simulink model "Virtual_Exhaust_Aftertreatment_Controller"  (R2016b)
settings: Solver=FixedStepDiscrete  StartTime=0.0  StopTime=inf  FixedStep=VirtExhATCtrlr.tiSimnTiStep_C  RelTol=1e-3  EnableMultiTasking=on
settings Model: Creator=m01wolf  LastModifiedBy=bunver
settings DataIOCC: SaveFormat=StructureWithTime  SaveOutput=off  DSMLogging=off  VisualizeSimOutput=off  SaveTime=off  SignalLoggingName=Results
settings OptimizationCC: BlockReduction=off  ConditionallyExecuteInputs=off  LifeSpan=inf
settings DebuggingCC: AllowSymbolicDim=off  SFUnexpectedBacktrackingDiag=warning  SFNoUnconditionalDefaultTransitionDiag=warning  SFExecutionAtInitializationDiag=none
settings ModelReferenceCC: ModelReferenceNumInstancesAllowed=Single  PropagateSignalLabelsOutOfModel=off
settings GRTTargetCC: TargetLangStandard=C89/C90 (ANSI)
settings ConfigComp: CovMetricSettings=dw  CovHtmlReporting=on  CovSaveCumulativeToWorkspaceVar=on  CovSaveSingleToWorkspaceVar=on  CovExternalEMLEnable=off

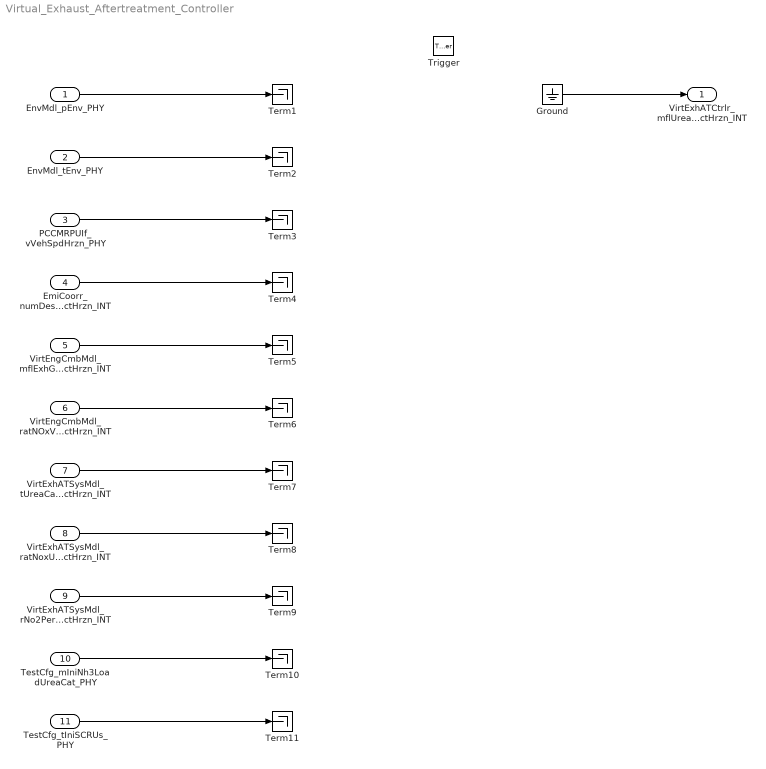
== system Virtual_Exhaust_Aftertreatment_Controller ==
  EnvMdl_pEnv_PHY : Inport
  EnvMdl_tEnv_PHY : Inport  Port=2
  PCCMRPUIf_vVehSpdHrzn_PHY : Inport  Port=3  PortDimensions=VirtExhATCtrlr_numHrznSize_CA
  EmiCoorr_numDesEngOperModVectHrzn_INT : Inport  Port=4  PortDimensions=VirtExhATCtrlr_numHrznSize_CA
  VirtEngCmbMdl_mflExhGasVectHrzn_INT : Inport  Port=5  PortDimensions=VirtExhATCtrlr_numHrznSize_CA
  VirtEngCmbMdl_ratNOxVectHrzn_INT : Inport  Port=6  PortDimensions=VirtExhATCtrlr_numHrznSize_CA
  VirtExhATSysMdl_tUreaCatUsVectHrzn_INT : Inport  Port=7  PortDimensions=VirtExhATCtrlr_numHrznSize_CA
  VirtExhATSysMdl_ratNoxUreaCatDsVectHrzn_INT : Inport  Port=8  PortDimensions=VirtExhATCtrlr_numHrznSize_CA
  VirtExhATSysMdl_rNo2PerNoxUreaCatUsVectHrzn_INT : Inport  Port=9  PortDimensions=VirtExhATCtrlr_numHrznSize_CA
  TestCfg_mIniNh3LoadUreaCat_PHY : Inport  Port=10
  TestCfg_tIniSCRUs_PHY : Inport  Port=11
  Trigger : TriggerPort  TriggerType=function-call  VariantControl=Variant  PortDimensions=1
  Ground : Ground
  Term{1..11} (11 alike) : Terminator
  VirtExhATCtrlr_mflUreaDesVectHrzn_INT : Outport  PortDimensions=VirtExhATCtrlr_numHrznSize_CA
  wires:
  Ground/1 -> VirtExhATCtrlr_mflUreaDesVectHrzn_INT/1
  EnvMdl_pEnv_PHY/1 -> Term1/1
  EnvMdl_tEnv_PHY/1 -> Term2/1
  VirtEngCmbMdl_mflExhGasVectHrzn_INT/1 -> Term5/1
  VirtExhATSysMdl_ratNoxUreaCatDsVectHrzn_INT/1 -> Term8/1
  VirtExhATSysMdl_rNo2PerNoxUreaCatUsVectHrzn_INT/1 -> Term9/1
  TestCfg_mIniNh3LoadUreaCat_PHY/1 -> Term10/1
  TestCfg_tIniSCRUs_PHY/1 -> Term11/1
  PCCMRPUIf_vVehSpdHrzn_PHY/1 -> Term3/1
  EmiCoorr_numDesEngOperModVectHrzn_INT/1 -> Term4/1
  VirtExhATSysMdl_tUreaCatUsVectHrzn_INT/1 -> Term7/1
  VirtEngCmbMdl_ratNOxVectHrzn_INT/1 -> Term6/1
